simulink subsystem "Vehicle1D_refsub_Driveline_withRoadProfile"  (R2022a)
settings: Solver=VariableStepAuto  StartTime=0.0  StopTime=10.0  RelTol=1e-3
undefined symbols (not defined in the file): vehicle
libraries: nesl_utility x10, fl_lib x4, sdl_lib x1
settings Model: Creator=isaacito  LastModifiedBy=isaacito
settings SolverCC: AlgebraicLoopSolver=TrustRegion
settings DebuggingCC: UnconnectedInputMsg=warning  UnconnectedOutputMsg=warning  UnconnectedLineMsg=warning  SFMachineParentedDataDiag=warning
settings RTWCC: DLArmComputeVersion=19.05

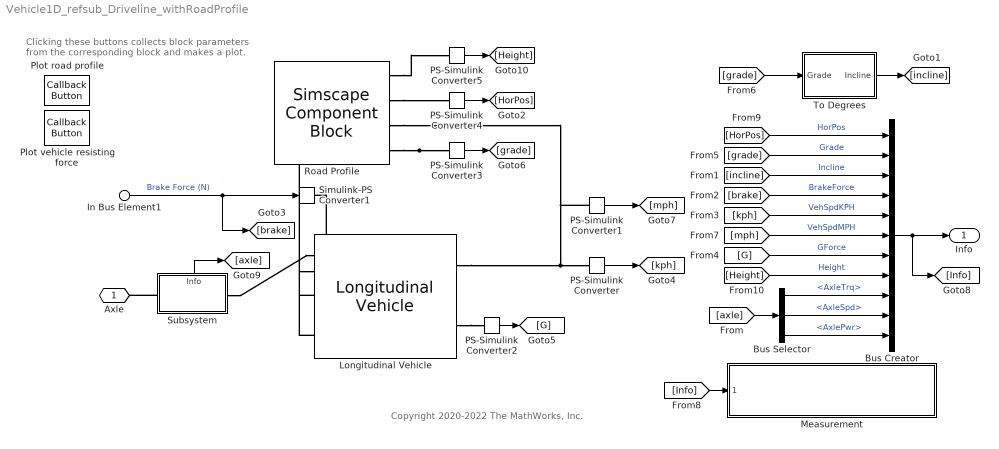
== system Vehicle1D_refsub_Driveline_withRoadProfile ==
  note: Clicking these buttons collects block parameters
      | from the corresponding block and makes a plot.
  note: Copyright 2020-2022 The MathWorks, Inc.
  In Bus Element1 : Inport  PortName=Inputs  Element=BrakeForce
      settings: AttributesFormatString=%<Unit>
  Bus Creator : BusCreator  Inputs=11
  Bus Selector : BusSelector  OutputSignals=AxleTrq,AxleSpd,AxlePwr
  Longitudinal Vehicle : sdl_lib/Tires & Vehicles/Longitudinal Vehicle  vehParamType=sdl.enum.VehicleParameterizationType.RoadLoad  M_vehicle=vehicle.mass_kg kg  R_tireroll=vehicle.tireRollingRadius_m m  C_tireroll=0.0136  C_airdrag=0.31  A_front=2.3 m^2  A_rl=vehicle.roadLoadA_N N  B_rl=vehicle.roadLoadB_N_per_kph N/(km/hr)  C_rl=vehicle.roadLoadC_N_per_kph2 N/(km/hr)^2  g=vehicle.roadLoad_gravAccel_m_per_s2 m/s^2  V_1=smoothing.vehicle_speedThreshold_kph km/hr  w_1=smoothing.vehicle_axleSpeedThreshold_rpm rpm  ShowBrakeIn=simscape.enum.onoff.on  ShowSlopeIn=simscape.enum.onoff.on  SlopeInputType=sdl.enum.VehicleLongitudinalRoadSlopeInputType.Grade  ShowWindIn=simscape.enum.onoff.off  ShowGOut=simscape.enum.onoff.on  air_density=1.184 kg/m^3  V_x_specify=on  V_x_priority=High  V_x=initial.vehicle_speed_kph km/hr  V_x_nominal_specify=off  V_x_nominal_unit=m/s  V_x_nominal_value=1  trq_specify=off  trq_priority=None  trq=0 N*m  trq_nominal_specify=off  trq_nominal_unit=N*m  trq_nominal_value=1  w_specify=off  w_priority=None  w=0 rad/s  w_nominal_specify=off  w_nominal_unit=rad/s  w_nominal_value=1
      settings: SourceProductBaseCode=LD  InternalSimscapePortConfiguration="{\"Bottom\":[],\"Left\":[{\"id\":\"Axle\",\"label\":\"Axle\",\"type\":\"foundation.mechanical.rotational.rotational\"}],\"Right\":[{\"id\":\"v_out\",\"label\":\"VehSpd\",\"type\":\"output\"},{\"id\":\"G_out\",\"label\":\"G\",\"type\":\"output\"}],\"Top\":[{\"id\":\"brkF\",\"label\":\"Brake\",\"type\":\"input\"},{\"id\":\"grade_norm\",\"label\":\"Grade\",\"type\":\"input\"}]}"
      settings: AttributesFormatString=|
      | Initial: %<V_x> [%<V_x_unit>]
      | Priority: %<V_x_priority>
  Measurement : Subsystem  ReferencedSubsystem=Vehicle1D_measurement_refsub_logging
  PS-Simulink Converter : nesl_utility/PS-Simulink Converter  PhysicalDomain=network_engine_domain  SubClassName=ps_output  LeftPortType=input  RightPortType=output  PseudoPeriodic=off  Frequencies=[]  VectorFormat=1-D array  Unit=km/hr  AffineConversion=off
      settings: SourceProductBaseCode=SS,PW,VE
  PS-Simulink Converter1 : nesl_utility/PS-Simulink Converter  PhysicalDomain=network_engine_domain  SubClassName=ps_output  LeftPortType=input  RightPortType=output  PseudoPeriodic=off  Frequencies=[]  VectorFormat=1-D array  Unit=mph  AffineConversion=off
      settings: SourceProductBaseCode=SS,PW,VE
  PS-Simulink Converter2 : nesl_utility/PS-Simulink Converter  PhysicalDomain=network_engine_domain  SubClassName=ps_output  LeftPortType=input  RightPortType=output  PseudoPeriodic=off  Frequencies=[]  VectorFormat=1-D array  Unit=1  AffineConversion=off
      settings: SourceProductBaseCode=SS,PW,VE
  PS-Simulink Converter3 : nesl_utility/PS-Simulink Converter  PhysicalDomain=network_engine_domain  SubClassName=ps_output  LeftPortType=input  RightPortType=output  PseudoPeriodic=off  Frequencies=[]  VectorFormat=1-D array  Unit=1  AffineConversion=off
      settings: SourceProductBaseCode=SS,PW,VE
  PS-Simulink Converter4 : nesl_utility/PS-Simulink Converter  PhysicalDomain=network_engine_domain  SubClassName=ps_output  LeftPortType=input  RightPortType=output  PseudoPeriodic=off  Frequencies=[]  VectorFormat=1-D array  Unit=m  AffineConversion=off
      settings: SourceProductBaseCode=SS,PW,VE
  PS-Simulink Converter5 : nesl_utility/PS-Simulink Converter  PhysicalDomain=network_engine_domain  SubClassName=ps_output  LeftPortType=input  RightPortType=output  PseudoPeriodic=off  Frequencies=[]  VectorFormat=1-D array  Unit=m  AffineConversion=off
      settings: SourceProductBaseCode=SS,PW,VE
  Plot road profile : CallbackButton  ButtonText=Plot
      settings: ClickFcn=|
      | % Select the block.
      | set_param(gcs, CurrentBlock="Road Profile")
      | 
      | plotRoadProfile(gcbh);
  Plot vehicle resisting force : CallbackButton  ButtonText=Plot
      settings: ClickFcn=|
      | % Select the block.
      | set_param(gcs, CurrentBlock="Longitudinal Vehicle")
      | 
      | Vehicle1D_plotProperties_Driveline(gcbh);
  Road Profile : SimscapeComponentBlock  SourceFile=RoadProfile1D_Custom  ComponentPath=RoadProfile1D_Custom  ComponentVariants="[\"RoadProfile1D_Custom\"]"  ComponentVariantNames="[\"RoadProfile1D_Custom\"]"  ClassName=RoadProfile1D_Custom  SchemaVersion=1  horizontalPosVec=road.HorizontalDistanceVec_m m  heightVec=road.VerticalProfileVec_m m  wheelbase=road.vehicleWheelbase_mm mm  x_specify=on  x_priority=High  x=initial.road_vehicleHorizontalPosition_m m  x_nominal_specify=off  x_nominal_unit=m  x_nominal_value=1
      settings: CopyFcn=simscape.engine.sli.internal.componentblockcallback(gcbh,'COPY')  PreCopyFcn=simscape.engine.sli.internal.componentblockcallback(gcbh,'PRECOPY')  PreDeleteFcn=simscape.engine.sli.internal.componentblockcallback(gcbh,'PREDELETE')  InternalSimscapePortConfiguration="{\"Bottom\":[],\"Left\":[],\"Right\":[{\"id\":\"z_out\",\"label\":\"Z\",\"type\":\"output\"},{\"id\":\"x_out\",\"label\":\"X\",\"type\":\"output\"},{\"id\":\"S\",\"label\":\"Spd\",\"type\":\"input\"},{\"id\":\"grade_norm\",\"label\":\"Gr\",\"type\":\"output\"}],\"Top\":[]}"
      mask Type: Simple Road Grade Profile
  Simulink-PS Converter1 : nesl_utility/Simulink-PS Converter  PhysicalDomain=network_engine_domain  SubClassName=ps_input  LeftPortType=input  RightPortType=output  PseudoPeriodic=off  Frequencies=[]  NoiseDistribution=none  NoiseParameters=[]  Unit=N  AffineConversion=off  FilteringAndDerivatives=filter  SimscapeFilterOrder=1  InputFilterTimeConstant=0.001  UdotUserProvided=0
      settings: SourceProductBaseCode=SS,PW,VE
  Subsystem : Subsystem
      settings: PortSchema="{\"entries\":[{\"content\":{\"sides\":[{\"content\":{\"connectorIds\":[\"LConn1\"]},\"type\":\"ConnectorPlacement.EquallySpacedRectSide\",\"uuid\":\"ec3cd8f6-c333-4ae9-94e8-194dcd7a9a9d\"},{\"content\":{\"connectorIds\":[\"RConn1\"],\"side\":\"RIGHT\"},\"type\":\"ConnectorPlacement.EquallySpacedRectSide\",\"uuid\":\"fef4b050-361f-4de4-b245-db8f722dbe30\"},{\"content\":{\"connectorIds\":[\"Out1\"],\"side\":\"TOP\"},\"type\":\"ConnectorPlacement.EquallySpacedRectSide\",\"uuid\":\"eda11c3e-d822-4525-9660-298bf232b628\"}]},\"type\":\"ConnectorPlacement.EquallySpacedConnector\",\"uuid\":\"afcb7fc3-0a34-49fa-b864-b9b6e2272b9d\"}],\"packageUris\":[\"http://schema.mathworks.com/mf0/Connector/R2020b\"],\"version\":\"1.0\"}"
  To Degrees : Subsystem
  Axle : PMIOPort  Side=Left
  Info : Outport
  wires:
  PS-Simulink Converter/1 -> [kph]
  PS-Simulink Converter2/1 -> [G]
  In Bus Element1/1 -> [brake], Simulink-PS Converter1/1  "Brake Force (N)"
  PS-Simulink Converter3/1 -> [grade]
  PS-Simulink Converter1/1 -> [mph]
  To Degrees/1(Incline) -> [incline]
  [grade] -> To Degrees/1(Grade)
  [grade] -> Bus Creator/2  "Grade"
  [incline] -> Bus Creator/3  "Incline"
  [brake] -> Bus Creator/4  "BrakeForce"
  Bus Creator/1 -> [Info], Info/1
  [Info] -> Measurement/1
  Subsystem/1(Info) -> [axle]
  [kph] -> Bus Creator/5  "VehSpdKPH"
  [mph] -> Bus Creator/6  "VehSpdMPH"
  [G] -> Bus Creator/7  "GForce"
  [axle] -> Bus Selector/1
  [HorPos] -> Bus Creator/1  "HorPos"
  PS-Simulink Converter4/1 -> [HorPos]
  PS-Simulink Converter5/1 -> [Height]
  Bus Selector/1 -> Bus Creator/9  "<AxleTrq>"
  Bus Selector/3 -> Bus Creator/11  "<AxlePwr>"
  [Height] -> Bus Creator/8  "Height"
  Bus Selector/2 -> Bus Creator/10  "<AxleSpd>"
  connections:
  Longitudinal Vehicle/RConn1 -- PS-Simulink Converter1/LConn1 -- Road Profile/RConn3 -- PS-Simulink Converter/LConn1
  Road Profile/RConn4 -- PS-Simulink Converter3/LConn1 -- Longitudinal Vehicle/LConn3
  Subsystem/LConn1 -- Axle/RConn1
  Longitudinal Vehicle/RConn2 -- PS-Simulink Converter2/LConn1
  Longitudinal Vehicle/LConn2 -- Simulink-PS Converter1/RConn1
  Subsystem/RConn1 -- Longitudinal Vehicle/LConn1
  Road Profile/RConn2 -- PS-Simulink Converter4/LConn1
  Road Profile/RConn1 -- PS-Simulink Converter5/LConn1

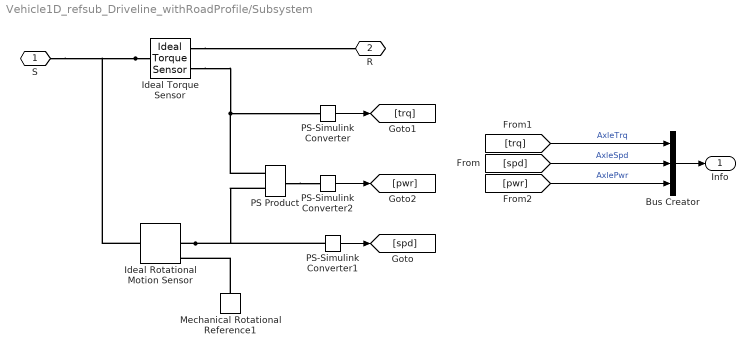
== system Vehicle1D_refsub_Driveline_withRoadProfile/Subsystem ==
  Bus Creator : BusCreator  Inputs=3
  Ideal Rotational Motion Sensor : fl_lib/Mechanical/Mechanical Sensors/Ideal Rotational Motion Sensor  wrap_angle=simscape.enum.onoff.off  offset=0 rad
      settings: SourceProductBaseCode=PW,SS,VE
  Ideal Torque Sensor : fl_lib/Mechanical/Mechanical Sensors/Ideal Torque Sensor
      settings: SourceProductBaseCode=PW,SS,VE
  Mechanical Rotational Reference1 : fl_lib/Mechanical/Rotational Elements/Mechanical Rotational Reference
      settings: SourceProductBaseCode=PW,SS,VE
  PS Product : fl_lib/Physical Signals/Functions/PS Product
      settings: SourceProductBaseCode=PW,SS,VE
  PS-Simulink Converter : nesl_utility/PS-Simulink Converter  PhysicalDomain=network_engine_domain  SubClassName=ps_output  LeftPortType=input  RightPortType=output  PseudoPeriodic=off  Frequencies=[]  VectorFormat=inherit  Unit=N*m  AffineConversion=off
      settings: SourceProductBaseCode=SS,PW,VE
  PS-Simulink Converter1 : nesl_utility/PS-Simulink Converter  PhysicalDomain=network_engine_domain  SubClassName=ps_output  LeftPortType=input  RightPortType=output  PseudoPeriodic=off  Frequencies=[]  VectorFormat=1-D array  Unit=rpm  AffineConversion=off
      settings: SourceProductBaseCode=SS,PW,VE
  PS-Simulink Converter2 : nesl_utility/PS-Simulink Converter  PhysicalDomain=network_engine_domain  SubClassName=ps_output  LeftPortType=input  RightPortType=output  PseudoPeriodic=off  Frequencies=[]  VectorFormat=inherit  Unit=kW  AffineConversion=off
      settings: SourceProductBaseCode=SS,PW,VE
  S : PMIOPort  Side=Left
  R : PMIOPort  Port=2  Side=Right
  Info : Outport
  wires:
  PS-Simulink Converter1/1 -> [spd]
  PS-Simulink Converter/1 -> [trq]
  PS-Simulink Converter2/1 -> [pwr]
  [trq] -> Bus Creator/1  "AxleTrq"
  [spd] -> Bus Creator/2  "AxleSpd"
  [pwr] -> Bus Creator/3  "AxlePwr"
  Bus Creator/1 -> Info/1
  connections:
  Mechanical Rotational Reference1/LConn1 -- Ideal Rotational Motion Sensor/RConn1
  Ideal Rotational Motion Sensor/RConn2 -- PS-Simulink Converter1/LConn1 -- PS Product/LConn2
  Ideal Torque Sensor/LConn1 -- S/RConn1 -- Ideal Rotational Motion Sensor/LConn1
  Ideal Torque Sensor/RConn1 -- R/RConn1
  Ideal Torque Sensor/RConn2 -- PS-Simulink Converter/LConn1 -- PS Product/LConn1
  PS Product/RConn1 -- PS-Simulink Converter2/LConn1

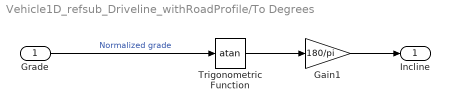
== system Vehicle1D_refsub_Driveline_withRoadProfile/To Degrees ==
  Grade : Inport  Unit=1
      settings: AttributesFormatString=%<Unit>
  Gain1 : Gain  Gain=180/pi
  Trigonometric Function : Trigonometry  Operator=atan
  Incline : Outport  Unit=deg
      settings: AttributesFormatString=%<Unit>
  wires:
  Gain1/1 -> Incline/1
  Trigonometric Function/1 -> Gain1/1
  Grade/1 -> Trigonometric Function/1  "Normalized grade"
